simulink model "sseg"  (Simulink 9.1)
settings: Solver=ode15s  StartTime=0.0  StopTime=Te  RelTol=1e-3  EnableMultiTasking=on
values from neighbouring files (symbols this model uses):
  A = [0 0 1 0;0 0 0 1;[d1w d2w d3w d4w]]    [fseg.m]
  B = [0 0;0 0;Ui]    [fseg.m]
  C = [1 1 0 0]    [butt.m]    (also in seg.m = [1 0 0 0])
  F = Fl2    [seg.m]
  xe = [0;pi/360;0;0]    [seg.m]
undefined symbols (not defined in the file or in its folder): D
libraries: cstblocks x1
settings Model: SuppressorTable=22 serialization::archive 11 0 6 0 0 0 1 0  Creator=cscherer  LastModifiedBy=nemezis
settings DataIOCC: LimitDataPoints=on  SignalLoggingSaveFormat=ModelDataLogs
settings OptimizationCC: ExpressionDepthLimit=2147483647  InitFltsAndDblsToZero=on
settings DebuggingCC: SaveWithParameterizedLinksMsg=none  SignalResolutionControl=TryResolveAllWithWarning  SolverPrmCheckMsg=warning  MultiTaskDSMMsg=warning  MultiTaskCondExecSysMsg=none  FcnCallInpInsideContextMsg=warning  StateNameClashWarn=warning
settings GRTTargetCC: TargetFcnLib=ansi_tfl_tmw.mat

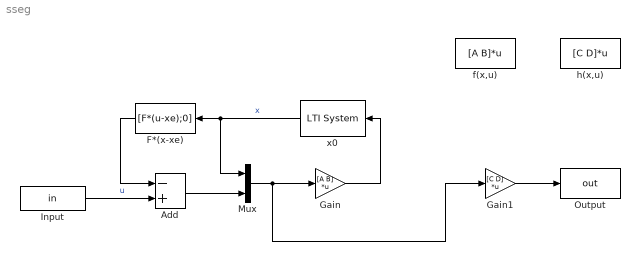
== system sseg ==
  Add : Sum  Inputs=-+
  F*(x-xe) : MATLABFcn  MATLABFcn=[F*(u-xe);0]
  Gain : Gain  Gain=[A B]  Multiplication=Matrix(K*u)
  Gain1 : Gain  Gain=[C D]  Multiplication=Matrix(K*u)
  Input : FromWorkspace  VariableName=in  SampleTime=0  OutputAfterFinalValue=Setting to zero
  Mux : Mux  Inputs=2
  Output : ToWorkspace  VariableName=out  SaveFormat=Structure With Time  SampleTime=-1
  f(x,u) : MATLABFcn  MATLABFcn=[A B]*u
  h(x,u) : MATLABFcn  MATLABFcn=[C D]*u
  x0 : cstblocks/LTI System  sys=integrator  IC=x0
  wires:
  Mux/1 -> Gain/1, Gain1/1
  x0/1 -> Mux/1, F*(x-xe)/1  "x"
  Add/1 -> Mux/2
  Input/1 -> Add/2  "u"
  F*(x-xe)/1 -> Add/1
  Gain1/1 -> Output/1
  Gain/1 -> x0/1
